simulink model "dc_motor_open_loop"  (R2024a)
settings: Solver=VariableStepAuto  StartTime=0.0  StopTime=10  RelTol=1e-3
undefined symbols (not defined in the file): B, J, Ke, Kt, L, R, TL
libraries: slpidlib x1
settings Model: Creator=27165  LastModifiedBy=27165

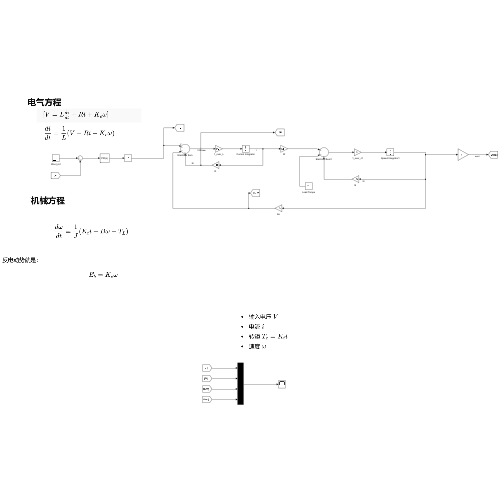
[thumbnail: Simulink's stored preview of the top-level diagram]
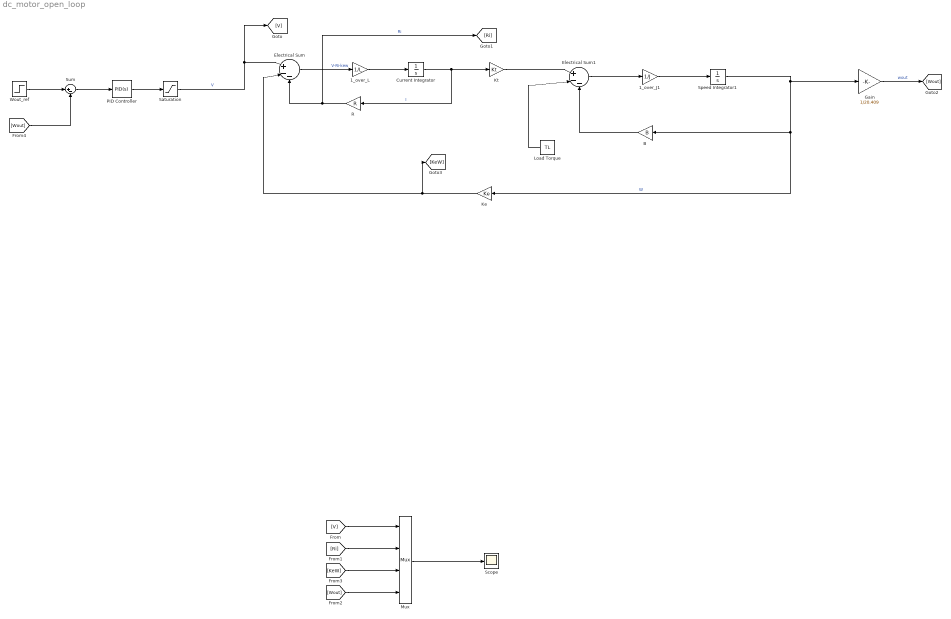
== system dc_motor_open_loop ==
  1_over_J1 : Gain  Gain=1/J
  1_over_L : Gain  Gain=1/L
  B : Gain  Gain=B
  Current Integrator : Integrator
  Electrical Sum : Sum  Inputs=|+--
  Electrical Sum1 : Sum  Inputs=|+--
  Gain : Gain  Gain=1/20.409
  Ke : Gain  Gain=Ke
  Kt : Gain  Gain=Kt
  Load Torque : Constant  Value=TL
  Mux : Mux
  PID Controller : slpidlib/PID Controller  Controller=PID  Form=Parallel  TimeDomain=Continuous-time  UseExternalTs=off  SampleTime=-1  IntegratorMethod=Forward Euler  FilterMethod=Forward Euler  ControllerParametersSource=internal  P=0.36  I=5.6  UseKiTs=off  D=0  UseExternalDerivativeSource=off  N=100  UseFilter=on  TunerSelectOption=Transfer Function Based (PID Tuner App)  InitialConditionSource=internal  InitialConditionForIntegrator=0  InitialConditionForFilter=0  DifferentiatorICPrevScaledInput=0  ExternalReset=none  TrackingMode=off  Kt=1  LimitOutput=off  SatLimitsSource=internal  UpperSaturationLimit=inf  LowerSaturationLimit=-inf  LinearizeAsGain=on  AntiWindupMode=none  Kb=1  LimitIntegrator=off  UpperIntegratorSaturationLimit=inf  LowerIntegratorSaturationLimit=-inf  POutMin=[]  POutMax=[]  IOutMin=[]  IOutMax=[]  DOutMin=[]  DOutMax=[]  NOutMin=[]  NOutMax=[]  SumOutMin=[]  SumOutMax=[]  SaturationOutMin=[]  SaturationOutMax=[]  PParamMin=[]  PParamMax=[]  IParamMin=[]  IParamMax=[]  DParamMin=[]  DParamMax=[]  NParamMin=[]  NParamMax=[]  KbParamMin=[]  KbParamMax=[]  KtParamMin=[]  KtParamMax=[]  KbOutMin=[]  KbOutMax=[]  KtOutMin=[]  KtOutMax=[]  IntegratorOutMin=[]  IntegratorOutMax=[]  FilterOutMin=[]  FilterOutMax=[]  SumI1OutMin=[]  SumI1OutMax=[]  SumI2OutMin=[]  SumI2OutMax=[]  SumI3OutMin=[]  SumI3OutMax=[]  SumI4OutMin=[]  SumI4OutMax=[]  SumDOutMin=[]  SumDOutMax=[]  DifferentiatorOutMin=[]  DifferentiatorOutMax=[]  FilterDiffOutCoefMin=[]  FilterDiffOutCoefMax=[]  ReciprocalOutMin=[]  ReciprocalOutMax=[]  SumDenOutMin=[]  SumDenOutMax=[]  SumNumOutMin=[]  SumNumOutMax=[]  DivideOutMin=[]  DivideOutMax=[]  UdiffTsProdOutMin=[]  UdiffTsProdOutMax=[]  NTsProdOutMin=[]  NTsProdOutMax=[]  UintegralTsProdOutMin=[]  UintegralTsProdOutMax=[]  UngainTsProdOutMin=[]  UngainTsProdOutMax=[]  ClampingZeroOutDataTypeStr=Inherit: Inherit via back propagation  ClampingZeroOutMin=[]  ClampingZeroOutMax=[]  FilterDenConstantOutDataTypeStr=Inherit: Inherit via back propagation  FilterDenConstantOutMin=[]  FilterDenConstantOutMax=[]  PCopyOutDataTypeStr=Inherit: Inherit via back propagation  PCopyOutMin=[]  PCopyOutMax=[]  NCopyOutDataTypeStr=Inherit: Inherit via back propagation  NCopyOutMin=[]  NCopyOutMax=[]  IntegratorContinuousStateAttributes=''  IntegratorStateMustResolveToSignalObject=off  IntegratorRTWStateStorageClass=Auto  FilterContinuousStateAttributes=''  FilterStateMustResolveToSignalObject=off  FilterRTWStateStorageClass=Auto  ParallelPVariant=InternalParameters  IdealPVariant=Disabled  IVariant=InternalParameters  DVariant=InternalParameters  IntegratorVariant=Continuous  SatVariant=Disabled  AWVariant=Passthrough  PCopyVariant=Disabled  TRVariant=Disabled  FdbkBlocksVariant=Forward  IdealPFdbkVariant=Disabled  SatFdbkVariant=Disabled  DerivativeFilterVariant=ContFilter  NVariant=InternalParameters  NCopyVariant=Disabled  FilterICVariant=InternalICsFilter  IntegratorICVariant=InternalICs  ExternalResetVariant=Disabled  TRSumVariant=Passthrough  SumFdbkVariant=Disabled  SumVariant=Sum_PID  TsampFilterVariant=InternalTs  TsampNgainVariant=Passthrough  TsampIntegralVariant=Disabled_SignalSpec  ExternalSaturationOutDataTypeStr=Inherit: Same as second input  DerivativeSourceVariant=ErrorSignal
  R : Gain  Gain=R
  Saturation : Saturate  UpperLimit=7.4  LowerLimit=-7.4
  Scope : Scope
  Speed Integrator1 : Integrator
  Sum : Sum  Inputs=|+-
  Wout_ref : Step  After=7  SampleTime=0
  wires:
  Saturation/1 -> [V], Electrical Sum/1  "V"
  Electrical Sum/1 -> 1_over_L/1  "V-Ri-kew"
  1_over_L/1 -> Current Integrator/1
  Current Integrator/1 -> Kt/1, R/1  "I"
  R/1 -> [Ri], Electrical Sum/3  "Ri"
  Ke/1 -> [KeW], Electrical Sum/2
  B/1 -> Electrical Sum1/3
  Electrical Sum1/1 -> 1_over_J1/1
  Speed Integrator1/1 -> Gain/1, Ke/1, B/1  "W"
  1_over_J1/1 -> Speed Integrator1/1
  Load Torque/1 -> Electrical Sum1/2
  Kt/1 -> Electrical Sum1/1
  Mux/1 -> Scope/1
  [V] -> Mux/1
  [Ri] -> Mux/2
  [Wout] -> Mux/4
  [KeW] -> Mux/3
  Gain/1 -> [Wout]  "wout"
  PID Controller/1 -> Saturation/1
  Sum/1 -> PID Controller/1
  Wout_ref/1 -> Sum/1
  [Wout] -> Sum/2
